simulink model "friction_model"  (R2016b)
settings: Solver=FixedStepAuto  StartTime=0.0  StopTime=H  FixedStep=h  RelTol=1e-3
values from neighbouring files (symbols this model uses):
  A = -0.6067    [initialize_friction_model.m]    (also in motor.m; run_motor.m)
  B = 0.8362    [initialize_friction_model.m]    (also in motor.m; run_motor.m)
  Cn = 65.3540    (= 65.354)    [initialize_friction_model.m]    (also in motor.m = 92.501; run_motor.m)
  Cst = C    (= 7)    [initialize_friction_model.m]
  Ct = 27.3769    [initialize_friction_model.m]    (also in motor.m; run_motor.m)
  F_load = 0    [initialize_friction_model.m]    (also in motor.m = 2; run_motor.m)
  Fp = 80    [initialize_friction_model.m]    (also in motor.m = 50; run_motor.m)
  Kn = 1.24E+09    (= 1240000000)    [initialize_friction_model.m]    (also in motor.m; run_motor.m)
  Kt = 557612763    [initialize_friction_model.m]    (also in motor.m; run_motor.m)
  Mn = 2.04E-02    (= 0.0204)    [initialize_friction_model.m]    (also in motor.m; run_motor.m)
  Mst = M    (= 0.18)    [initialize_friction_model.m]
  Mt = 9.33E-03    (= 0.00933)    [initialize_friction_model.m]    (also in motor.m; run_motor.m)
  mu = 0.35    [initialize_friction_model.m]    (also in motor.m; run_motor.m)
  mu_s = 0.001    [initialize_friction_model.m]    (also in motor.m; run_motor.m)
  Nst = 0    [initialize_friction_model.m]
  phi = alpha    (= 1.57079632679)    [initialize_friction_model.m]
  ws = 2*pi*fs    (= 245044.22698)    [initialize_friction_model.m]    (also in motor.m; run_motor.m)
settings Model: Creator=admin  LastModifiedBy=admin

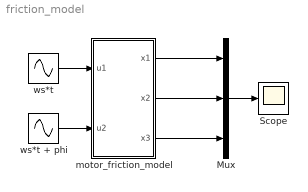
== system friction_model ==
  Mux : Mux  Inputs=3
  Scope : Scope
  motor_friction_model : Subsystem
  ws*t : Sin  Frequency=ws  SampleTime=0
  ws*t + phi : Sin  Frequency=ws  Phase=phi  SampleTime=0
  wires:
  ws*t/1 -> motor_friction_model/1(u1)
  motor_friction_model/1(x1) -> Mux/1
  motor_friction_model/2(x2) -> Mux/2
  motor_friction_model/3(x3) -> Mux/3
  Mux/1 -> Scope/1
  ws*t + phi/1 -> motor_friction_model/2(u2)

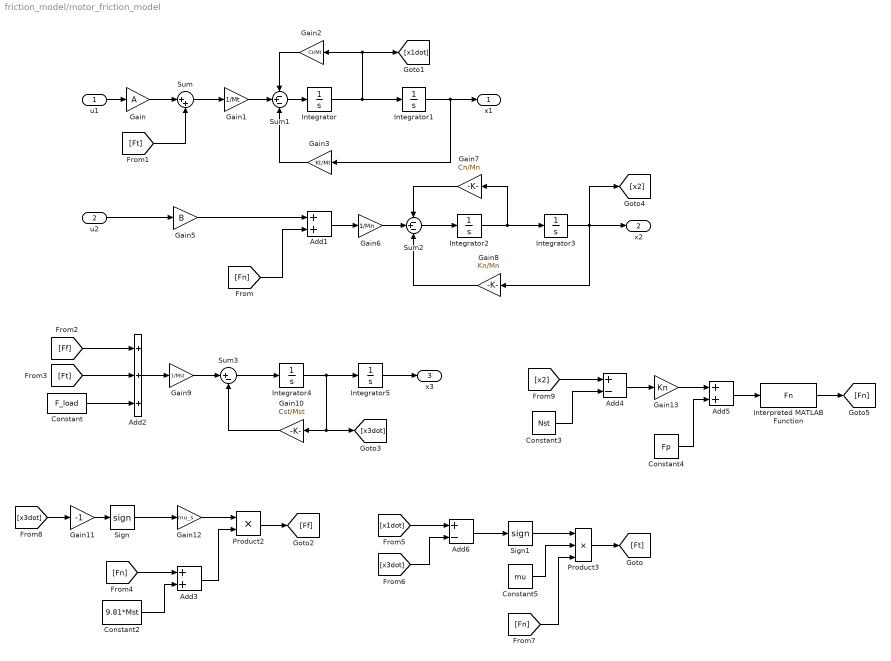
== system friction_model/motor_friction_model ==
  u1 : Inport
  u2 : Inport  Port=2
  Add1 : Sum
  Add2 : Sum  Inputs=3
  Add3 : Sum
  Add4 : Sum  Inputs=+-
  Add5 : Sum
  Add6 : Sum  Inputs=+-
  Constant : Constant  Value=F_load
  Constant2 : Constant  Value=9.81*Mst
  Constant3 : Constant  Value=Nst
  Constant4 : Constant  Value=Fp
  Constant5 : Constant  Value=mu
  Gain : Gain  Gain=A
  Gain1 : Gain  Gain=1/Mt
  Gain10 : Gain  Gain=Cst/Mst
  Gain11 : Gain  Gain=-1
  Gain12 : Gain  Gain=mu_s
  Gain13 : Gain  Gain=Kn
  Gain2 : Gain  Gain=Ct/Mt
  Gain3 : Gain  Gain=Kt/Mt
  Gain5 : Gain  Gain=B
  Gain6 : Gain  Gain=1/Mn
  Gain7 : Gain  Gain=Cn/Mn
  Gain8 : Gain  Gain=Kn/Mn
  Gain9 : Gain  Gain=1/Mst
  Integrator{,1..5} (6 alike) : Integrator
  Interpreted MATLAB Function : MATLABFcn  MATLABFcn=Fn  OutputDimensions=1
  Product2 : Product
  Product3 : Product  Inputs=3
  Sign : Signum
  Sign1 : Signum
  Sum : Sum  Inputs=|++
  Sum1 : Sum  Inputs=-+-
  Sum2 : Sum  Inputs=-+-
  Sum3 : Sum  Inputs=|+-
  x1 : Outport
  x2 : Outport  Port=2
  x3 : Outport  Port=3
  wires:
  Gain/1 -> Sum/1
  [Ft] -> Sum/2
  Sum/1 -> Gain1/1
  Gain1/1 -> Sum1/2
  Sum1/1 -> Integrator/1
  Integrator/1 -> [x1dot], Gain2/1, Integrator1/1
  Gain2/1 -> Sum1/1
  Integrator1/1 -> Gain3/1, x1/1
  Gain3/1 -> Sum1/3
  Gain5/1 -> Add1/1
  [Fn] -> Add1/2
  Add1/1 -> Gain6/1
  Gain6/1 -> Sum2/2
  Sum2/1 -> Integrator2/1
  Integrator2/1 -> Gain7/1, Integrator3/1
  Gain7/1 -> Sum2/1
  Integrator3/1 -> [x2], Gain8/1, x2/1
  Gain8/1 -> Sum2/3
  [Ff] -> Add2/1
  [Ft] -> Add2/2
  Constant/1 -> Add2/3
  Add2/1 -> Gain9/1
  Gain9/1 -> Sum3/1
  Sum3/1 -> Integrator4/1
  Gain10/1 -> Sum3/2
  Integrator5/1 -> x3/1
  Gain11/1 -> Sign/1
  Sign/1 -> Gain12/1
  Gain12/1 -> Product2/1
  Add3/1 -> Product2/2
  [Fn] -> Add3/1
  Constant2/1 -> Add3/2
  Product2/1 -> [Ff]
  Constant3/1 -> Add4/2
  Add4/1 -> Gain13/1
  Gain13/1 -> Add5/1
  Constant4/1 -> Add5/2
  Integrator4/1 -> [x3dot], Gain10/1, Integrator5/1
  [x1dot] -> Add6/1
  [x3dot] -> Add6/2
  Add6/1 -> Sign1/1
  Sign1/1 -> Product3/1
  Constant5/1 -> Product3/2
  [Fn] -> Product3/3
  Product3/1 -> [Ft]
  [x3dot] -> Gain11/1
  [x2] -> Add4/1
  Add5/1 -> Interpreted MATLAB Function/1
  Interpreted MATLAB Function/1 -> [Fn]
  u2/1 -> Gain5/1
  u1/1 -> Gain/1
